simulink model "snap2_f_200msps_64i_4096c"  (R2019a)
settings: Solver=VariableStepDiscrete  StartTime=0.0  StopTime=10.0  RelTol=1e-3
undefined symbols (not defined in the file or in its folder): datetime, posixtime
libraries: xbsIndex_r4 x21354, casper_library_misc x297, casper_library_delays x19, xps_library x14, casper_library_sources x4
(part 28 of 217)

== system snap2_f_200msps_64i_4096c/input/rms ==
  note: two clocks after
      | adc_rms_rst goes high
      | the outputs are locked
  note: To provide a means for measuring the magnitude of the signals
      | coming in to each ADC channel, we have a "calc_adc_sum_sq"
      | block which uses a single multiplier, two accumulators, and two
      | regsiters to calculate the sum of 64K ADC samples and the sum
      | of squares of 64K ADC samples.  These can be used to calculate
      | the mean (aka DC offset) and standard deviation (aka RMS) of
      | the ADC inputs.
  note: The sum_sumsq values are Fix_64_0.
      | The upper 29 bits are Fix_29_0 sum of samples.
      | The lower 35 bits are UFix_35_0 sum of squares.
  note: sum,sq,sum,sq,...
  in : Inport
  Constant : Constant  Value=0
  Counter : xbsIndex_r4/Counter  cnt_type=Free Running  cnt_to=Inf  operation=Up  start_count=0  cnt_by_val=1  arith_type=Unsigned  n_bits=16  bin_pt=0  load_pin=off  rst=off  en=off  explicit_period=off  period=1  use_behavioral_HDL=off  implementation=Fabric  use_rpm=on  dbl_ovrd=off  block_type=counter
      settings: xl_area=[0, 0, 0, 0, 0, 0, 0]
  Slice16 : xbsIndex_r4/Slice  nbits=1  boolean_output=on  mode=Upper Bit Location + Width  bit1=0  base1=MSB of Input  bit0=19  base0=LSB of Input  dbl_ovrd=off  block_type=slice
      settings: infoedit="Extracts a given range of bits from each input sample and presents it at the output.  The output type is ordinarily unsigned with binary point at zero, but can be Boolean when the slice is one bit wide.<P><P>Hardware notes: In hardware this block costs nothing."  block_version=10.1.3
  Terminator : Terminator
  bram_ctrl : Subsystem
  bus_expand : Subsystem  AncestorBlock=casper_library_flow_control/bus_expand  mask(bus_expand){mode=divisions of equal size, outputNum=64, outputWidth=10, outputBinaryPt=0, outputArithmeticType=1, show_format=off, outputToWorkspace=off, variablePrefix=out, outputToModelAsWell=on}
      mask prompts: outputNum "Number of outputs:"; outputWidth "Output width:"; outputBinaryPt "Output binary point position:"; outputArithmeticType "Output arithmetic type (ufix=0, fix=1, bool=2):"; show_format "Print format string?"; outputToWorkspace "Output to workspace?"; variablePrefix "Variable name prefix:"; outputToModelAsWell "Output to model as well?"
      mask help:
      | Expands a 'bus' made using a bus_create or Xilinx
      | concat block.
      | The input will be divided into the specified number
      | of outputs with the specified arithmetic types.
      | Divisions are made from most significant bit.
      mask init: same as snap2_f_200msps_64i_4096c/autocorr/bus_expand
      settings: AttributesFormatString=64 outputs
      mask TypeOptions mode: divisions of equal size | divisions of arbitrary size
      mask Callback mode: bus_expand_callback();
      mask Callback outputWidth: bus_expand_callback();
      mask Callback outputToWorkspace: bus_expand_callback();
  calc_adc_sum_sq0 : Subsystem
  calc_adc_sum_sq1 : Subsystem
  calc_adc_sum_sq10 : Subsystem
  calc_adc_sum_sq11 : Subsystem
  calc_adc_sum_sq12 : Subsystem
  calc_adc_sum_sq13 : Subsystem
  calc_adc_sum_sq14 : Subsystem
  calc_adc_sum_sq15 : Subsystem
  calc_adc_sum_sq16 : Subsystem
  calc_adc_sum_sq17 : Subsystem
  calc_adc_sum_sq18 : Subsystem
  calc_adc_sum_sq19 : Subsystem
  calc_adc_sum_sq2 : Subsystem
  calc_adc_sum_sq20 : Subsystem
  calc_adc_sum_sq21 : Subsystem
  calc_adc_sum_sq22 : Subsystem
  calc_adc_sum_sq23 : Subsystem
  calc_adc_sum_sq24 : Subsystem
  calc_adc_sum_sq25 : Subsystem
  calc_adc_sum_sq26 : Subsystem
  calc_adc_sum_sq27 : Subsystem
  calc_adc_sum_sq28 : Subsystem
  calc_adc_sum_sq29 : Subsystem
  calc_adc_sum_sq3 : Subsystem
  calc_adc_sum_sq30 : Subsystem
  calc_adc_sum_sq31 : Subsystem
  calc_adc_sum_sq32 : Subsystem
  calc_adc_sum_sq33 : Subsystem
  calc_adc_sum_sq34 : Subsystem
  calc_adc_sum_sq35 : Subsystem
  calc_adc_sum_sq36 : Subsystem
  calc_adc_sum_sq37 : Subsystem
  calc_adc_sum_sq38 : Subsystem
  calc_adc_sum_sq39 : Subsystem
  calc_adc_sum_sq4 : Subsystem
  calc_adc_sum_sq40 : Subsystem
  calc_adc_sum_sq41 : Subsystem
  calc_adc_sum_sq42 : Subsystem
  calc_adc_sum_sq43 : Subsystem
  calc_adc_sum_sq44 : Subsystem
  calc_adc_sum_sq45 : Subsystem
  calc_adc_sum_sq46 : Subsystem
  calc_adc_sum_sq47 : Subsystem
  calc_adc_sum_sq48 : Subsystem
  calc_adc_sum_sq49 : Subsystem
  calc_adc_sum_sq5 : Subsystem
  calc_adc_sum_sq50 : Subsystem
  calc_adc_sum_sq51 : Subsystem
  calc_adc_sum_sq52 : Subsystem
  calc_adc_sum_sq53 : Subsystem
  calc_adc_sum_sq54 : Subsystem
  calc_adc_sum_sq55 : Subsystem
  calc_adc_sum_sq56 : Subsystem
  calc_adc_sum_sq57 : Subsystem
  calc_adc_sum_sq58 : Subsystem
  calc_adc_sum_sq59 : Subsystem
  calc_adc_sum_sq6 : Subsystem
  calc_adc_sum_sq60 : Subsystem
  calc_adc_sum_sq61 : Subsystem
  calc_adc_sum_sq62 : Subsystem
  calc_adc_sum_sq63 : Subsystem
  calc_adc_sum_sq7 : Subsystem
  calc_adc_sum_sq8 : Subsystem
  calc_adc_sum_sq9 : Subsystem
  edge_detect : Subsystem  AncestorBlock=casper_library_misc/edge_detect  mask(edge_detect){edge=Rising, polarity=Active High, x_in=[0 0.08 0.08 0.16 0.16 0.24 0.24 0.32 0.32 0.4], y_in=[-1 -1  1  1  1  1  1  1  1  1], x_out=[0.6 0.68 0.68 0.76 0.76 0.84 0.84 0.92 0.92 1], y_out=[-1 -1  1  1 -1 -1 -1 -1 -1 -1]}
      mask prompts: edge "Edge Type"; polarity "Output Polarity"; x_in "Input X Positions"; y_in "Input Y Positions"; x_out "Output X Positions"; y_out "Output Y Positions"
      mask help: Output is active for one-cycle after each edge of the specified type (i.e. rising, falling or both).
      mask init: same as snap2_f_200msps_64i_4096c/cosmic_ray/edge_detect
      settings: AttributesFormatString=|
      | rising edges
      | active high
      mask Help: Output is active for one-cycle after each edge of the specified type (i.e. rising, falling, or both).  Latency is zero.
      mask TypeOptions edge: Rising | Falling | Both
      mask TypeOptions polarity: Active High | Active Low
      mask Display:
      | plot(x_in_num,0.5+y_in_num*0.2);
      | plot(x_out_num,0.5+y_out_num*0.2);
  enable : Subsystem  Tag=xps:sw_reg  AncestorBlock=xps_library/Memory/software_register  mask(swreg){io_dir=From Processor, io_delay=0, init_val=0, sample_period=1, names=reg, bitwidths=32, bin_pts=0, arith_types=0, sim_port=on, show_format=off, desc_str=|}
      mask desc_str=|
      | Enable statistics recording. If the least-significant bit
      | is ``1``, statistics will be recorded to RAM.
      mask prompts: io_dir "I/O direction"; io_delay "I/O delay"; init_val "Initial Value"; sample_period "Sample period"; names "Bitfield names [msb...lsb]"; bitwidths "Bitfield widths"; bin_pts "Bitfield binary pts"; arith_types "Bitfield types, ufix=0, fix=1, bool=2"; sim_port "Provide sim input/output?"; show_format "Print format string?"; desc_str "Description"
      mask help: A 32-bit software-accessible register. Can be divided into bitfields of varying widths and types using the fields in the block mask.
      mask init:
      | swreg_init(gcb)
      settings: AttributesFormatString=1input
      mask TypeOptions io_dir: To Processor | From Processor
      mask Callback io_dir:
      | mask_enables = get_param(gcb, 'MaskEnables');
      | mask_names = get_param(gcb, 'MaskNames');
      | if strcmp(get_param(gcb, 'io_dir'), 'To Processor'),
      |     mask_enables{ismember(mask_names, 'sample_period')} = 'off';
      | else
      |     mask_enables{ismember(mask_names, 'sample_period')} = 'on';
      | end
      | set_param(gcb, 'MaskEnables', mask_enables);
      mask DialogControl ParameterTabVar0 Prompt: Setup
  levels : Subsystem  Tag=xps:bram  AncestorBlock=xps_library/Memory/shared_bram  mask{sample_rate=1, init_vals=[0:2^10-1], data_bin_pt=0, optimization=Minimum_Area, reg_core_output=on, reg_prim_output=on, data_width=64, addr_width=9, arith_type=Unsigned, desc_str=|, type_desc=uint64}
      mask desc_str=|
      | Multi-channel statistics. For the ``n`` th 64-bit word, the
      | least signficant 32 bits represent the accumulated
      | ADC power, accumulated over 65536 samples and
      | stored as an unsigned 32-bit integer.
      | The most significant 32 bits represent the sum of
      | 65536 ADC samples stored as a signed 32-bit integer.
      mask prompts: sample_rate "Sample rate"; init_vals "Initial values (simulation only)"; data_bin_pt "Data Binary Point"; reg_core_output "Register Core Output"; reg_prim_output "Register Primitive Output"; data_width "Data Width"; addr_width "Address width"; arith_type "Output Data Type"; desc_str "Description"; type_desc "Word Type Description"
      mask init:
      | shared_bram_mask;
      mask TypeOptions optimization: Minimum_Area | Low_Power
      mask TypeOptions data_width: 8 | 16 | 32 | 64 | 128
      mask TypeOptions arith_type: Unsigned | Signed  (2's comp)
      mask DialogControl Container4 Prompt: Configuration
      mask DialogControl Container10 Prompt: Documentation
  lsb : xbsIndex_r4/Slice  nbits=0  boolean_output=on  mode=Lower Bit Location + Width  bit1=0  base1=MSB of Input  bit0=0  base0=LSB of Input  dbl_ovrd=off  block_type=slice
      settings: block_version=10.1.3
  tag scope: adc_rms_rst=global
  wires:
  Counter/1 -> Slice16/1
  Slice16/1 -> edge_detect/1(in)
  edge_detect/1(out) -> [adc_rms_rst]
  enable/1(in_reg) -> lsb/1
  bram_ctrl/1(addr) -> levels/1(addr)
  bram_ctrl/2(data) -> levels/2(data_in)
  bram_ctrl/3(we) -> levels/3(we)
  Constant/1 -> enable/1(sim_1)
  levels/1(data_out) -> Terminator/1
  in/1 -> bus_expand/1(bus_in)
  lsb/1 -> bram_ctrl/1(en)
  calc_adc_sum_sq36/1(sum_sumsq) -> bram_ctrl/46(adc44)
  calc_adc_sum_sq12/1(sum_sumsq) -> bram_ctrl/14(adc12)
  calc_adc_sum_sq30/1(sum_sumsq) -> bram_ctrl/26(adc24)
  calc_adc_sum_sq28/1(sum_sumsq) -> bram_ctrl/24(adc22)
  calc_adc_sum_sq58/1(sum_sumsq) -> bram_ctrl/38(adc36)
  calc_adc_sum_sq55/1(sum_sumsq) -> bram_ctrl/37(adc35)
  calc_adc_sum_sq18/1(sum_sumsq) -> bram_ctrl/28(adc26)
  calc_adc_sum_sq24/1(sum_sumsq) -> bram_ctrl/20(adc18)
  calc_adc_sum_sq22/1(sum_sumsq) -> bram_ctrl/32(adc30)
  calc_adc_sum_sq32/1(sum_sumsq) -> bram_ctrl/34(adc32)
  calc_adc_sum_sq25/1(sum_sumsq) -> bram_ctrl/21(adc19)
  calc_adc_sum_sq23/1(sum_sumsq) -> bram_ctrl/33(adc31)
  calc_adc_sum_sq31/1(sum_sumsq) -> bram_ctrl/27(adc25)
  calc_adc_sum_sq19/1(sum_sumsq) -> bram_ctrl/29(adc27)
  calc_adc_sum_sq13/1(sum_sumsq) -> bram_ctrl/15(adc13)
  calc_adc_sum_sq35/1(sum_sumsq) -> bram_ctrl/45(adc43)
  calc_adc_sum_sq39/1(sum_sumsq) -> bram_ctrl/49(adc47)
  calc_adc_sum_sq38/1(sum_sumsq) -> bram_ctrl/48(adc46)
  calc_adc_sum_sq57/1(sum_sumsq) -> bram_ctrl/59(adc57)
  calc_adc_sum_sq48/1(sum_sumsq) -> bram_ctrl/65(adc63)
  calc_adc_sum_sq16/1(sum_sumsq) -> bram_ctrl/18(adc16)
  calc_adc_sum_sq27/1(sum_sumsq) -> bram_ctrl/23(adc21)
  calc_adc_sum_sq50/1(sum_sumsq) -> bram_ctrl/53(adc51)
  calc_adc_sum_sq42/1(sum_sumsq) -> bram_ctrl/60(adc58)
  calc_adc_sum_sq15/1(sum_sumsq) -> bram_ctrl/17(adc15)
  calc_adc_sum_sq26/1(sum_sumsq) -> bram_ctrl/22(adc20)
  calc_adc_sum_sq49/1(sum_sumsq) -> bram_ctrl/52(adc50)
  calc_adc_sum_sq54/1(sum_sumsq) -> bram_ctrl/57(adc55)
  calc_adc_sum_sq51/1(sum_sumsq) -> bram_ctrl/54(adc52)
  calc_adc_sum_sq14/1(sum_sumsq) -> bram_ctrl/16(adc14)
  calc_adc_sum_sq20/1(sum_sumsq) -> bram_ctrl/30(adc28)
  calc_adc_sum_sq17/1(sum_sumsq) -> bram_ctrl/19(adc17)
  calc_adc_sum_sq33/1(sum_sumsq) -> bram_ctrl/35(adc33)
  calc_adc_sum_sq53/1(sum_sumsq) -> bram_ctrl/56(adc54)
  calc_adc_sum_sq21/1(sum_sumsq) -> bram_ctrl/31(adc29)
  calc_adc_sum_sq59/1(sum_sumsq) -> bram_ctrl/39(adc37)
  calc_adc_sum_sq47/1(sum_sumsq) -> bram_ctrl/64(adc62)
  calc_adc_sum_sq52/1(sum_sumsq) -> bram_ctrl/55(adc53)
  calc_adc_sum_sq61/1(sum_sumsq) -> bram_ctrl/41(adc39)
  calc_adc_sum_sq46/1(sum_sumsq) -> bram_ctrl/63(adc61)
  calc_adc_sum_sq34/1(sum_sumsq) -> bram_ctrl/44(adc42)
  calc_adc_sum_sq56/1(sum_sumsq) -> bram_ctrl/58(adc56)
  calc_adc_sum_sq60/1(sum_sumsq) -> bram_ctrl/40(adc38)
  calc_adc_sum_sq62/1(sum_sumsq) -> bram_ctrl/42(adc40)
  calc_adc_sum_sq29/1(sum_sumsq) -> bram_ctrl/25(adc23)
  calc_adc_sum_sq44/1(sum_sumsq) -> bram_ctrl/36(adc34)
  calc_adc_sum_sq41/1(sum_sumsq) -> bram_ctrl/51(adc49)
  calc_adc_sum_sq37/1(sum_sumsq) -> bram_ctrl/47(adc45)
  calc_adc_sum_sq43/1(sum_sumsq) -> bram_ctrl/61(adc59)
  calc_adc_sum_sq63/1(sum_sumsq) -> bram_ctrl/43(adc41)
  calc_adc_sum_sq40/1(sum_sumsq) -> bram_ctrl/50(adc48)
  calc_adc_sum_sq0/1(sum_sumsq) -> bram_ctrl/2(adc0)
  calc_adc_sum_sq1/1(sum_sumsq) -> bram_ctrl/3(adc1)
  calc_adc_sum_sq10/1(sum_sumsq) -> bram_ctrl/12(adc10)
  calc_adc_sum_sq11/1(sum_sumsq) -> bram_ctrl/13(adc11)
  calc_adc_sum_sq2/1(sum_sumsq) -> bram_ctrl/4(adc2)
  calc_adc_sum_sq3/1(sum_sumsq) -> bram_ctrl/5(adc3)
  calc_adc_sum_sq4/1(sum_sumsq) -> bram_ctrl/6(adc4)
  calc_adc_sum_sq5/1(sum_sumsq) -> bram_ctrl/7(adc5)
  calc_adc_sum_sq6/1(sum_sumsq) -> bram_ctrl/8(adc6)
  calc_adc_sum_sq7/1(sum_sumsq) -> bram_ctrl/9(adc7)
  calc_adc_sum_sq8/1(sum_sumsq) -> bram_ctrl/10(adc8)
  calc_adc_sum_sq9/1(sum_sumsq) -> bram_ctrl/11(adc9)
  calc_adc_sum_sq45/1(sum_sumsq) -> bram_ctrl/62(adc60)
  bus_expand/41(out24) -> calc_adc_sum_sq62/1(in)
  bus_expand/40(out25) -> calc_adc_sum_sq61/1(in)
  bus_expand/39(out26) -> calc_adc_sum_sq60/1(in)
  bus_expand/1(msb_out64) -> calc_adc_sum_sq0/1(in)
  bus_expand/2(out63) -> calc_adc_sum_sq1/1(in)
  bus_expand/45(out20) -> calc_adc_sum_sq36/1(in)
  bus_expand/30(out35) -> calc_adc_sum_sq21/1(in)
  bus_expand/33(out32) -> calc_adc_sum_sq32/1(in)
  bus_expand/52(out13) -> calc_adc_sum_sq50/1(in)
  bus_expand/35(out30) -> calc_adc_sum_sq44/1(in)
  bus_expand/51(out14) -> calc_adc_sum_sq49/1(in)
  bus_expand/49(out16) -> calc_adc_sum_sq40/1(in)
  bus_expand/44(out21) -> calc_adc_sum_sq35/1(in)
  bus_expand/53(out12) -> calc_adc_sum_sq51/1(in)
  bus_expand/5(out60) -> calc_adc_sum_sq4/1(in)
  bus_expand/7(out58) -> calc_adc_sum_sq6/1(in)
  bus_expand/4(out61) -> calc_adc_sum_sq3/1(in)
  bus_expand/37(out28) -> calc_adc_sum_sq58/1(in)
  bus_expand/9(out56) -> calc_adc_sum_sq8/1(in)
  bus_expand/10(out55) -> calc_adc_sum_sq9/1(in)
  bus_expand/11(out54) -> calc_adc_sum_sq10/1(in)
  bus_expand/34(out31) -> calc_adc_sum_sq33/1(in)
  bus_expand/36(out29) -> calc_adc_sum_sq55/1(in)
  bus_expand/48(out17) -> calc_adc_sum_sq39/1(in)
  bus_expand/29(out36) -> calc_adc_sum_sq20/1(in)
  bus_expand/47(out18) -> calc_adc_sum_sq38/1(in)
  bus_expand/31(out34) -> calc_adc_sum_sq22/1(in)
  bus_expand/43(out22) -> calc_adc_sum_sq34/1(in)
  bus_expand/50(out15) -> calc_adc_sum_sq41/1(in)
  bus_expand/46(out19) -> calc_adc_sum_sq37/1(in)
  bus_expand/38(out27) -> calc_adc_sum_sq59/1(in)
  bus_expand/17(out48) -> calc_adc_sum_sq16/1(in)
  bus_expand/13(out52) -> calc_adc_sum_sq12/1(in)
  bus_expand/14(out51) -> calc_adc_sum_sq13/1(in)
  bus_expand/15(out50) -> calc_adc_sum_sq14/1(in)
  bus_expand/16(out49) -> calc_adc_sum_sq15/1(in)
  bus_expand/18(out47) -> calc_adc_sum_sq17/1(in)
  bus_expand/19(out46) -> calc_adc_sum_sq24/1(in)
  bus_expand/20(out45) -> calc_adc_sum_sq25/1(in)
  bus_expand/21(out44) -> calc_adc_sum_sq26/1(in)
  bus_expand/22(out43) -> calc_adc_sum_sq27/1(in)
  bus_expand/23(out42) -> calc_adc_sum_sq28/1(in)
  bus_expand/24(out41) -> calc_adc_sum_sq29/1(in)
  bus_expand/25(out40) -> calc_adc_sum_sq30/1(in)
  bus_expand/26(out39) -> calc_adc_sum_sq31/1(in)
  bus_expand/27(out38) -> calc_adc_sum_sq18/1(in)
  bus_expand/28(out37) -> calc_adc_sum_sq19/1(in)
  bus_expand/3(out62) -> calc_adc_sum_sq2/1(in)
  bus_expand/8(out57) -> calc_adc_sum_sq7/1(in)
  bus_expand/12(out53) -> calc_adc_sum_sq11/1(in)
  bus_expand/6(out59) -> calc_adc_sum_sq5/1(in)
  bus_expand/42(out23) -> calc_adc_sum_sq63/1(in)
  bus_expand/32(out33) -> calc_adc_sum_sq23/1(in)
  bus_expand/54(out11) -> calc_adc_sum_sq52/1(in)
  bus_expand/55(out10) -> calc_adc_sum_sq53/1(in)
  bus_expand/56(out9) -> calc_adc_sum_sq54/1(in)
  bus_expand/57(out8) -> calc_adc_sum_sq56/1(in)
  bus_expand/58(out7) -> calc_adc_sum_sq57/1(in)
  bus_expand/59(out6) -> calc_adc_sum_sq42/1(in)
  bus_expand/60(out5) -> calc_adc_sum_sq43/1(in)
  bus_expand/61(out4) -> calc_adc_sum_sq45/1(in)
  bus_expand/62(out3) -> calc_adc_sum_sq46/1(in)
  bus_expand/63(out2) -> calc_adc_sum_sq47/1(in)
  bus_expand/64(lsb_out1) -> calc_adc_sum_sq48/1(in)

== system snap2_f_200msps_64i_4096c/input/source_sel0 ==
  sim_1 : Inport
  convert1_1 : DataTypeConversion  OutDataTypeStr=fixdt('ufix32_En0')  LockScale=on
  convert2_1 : DataTypeConversion  OutDataTypeStr=fixdt('ufix32_En0')  ConvertRealWorld=Stored Integer (SI)  LockScale=on
  gain_1 : Gain
  io_delay : xbsIndex_r4/Delay  rst=off  infoeditControl=Selection of Reset will increase slice count due to use of real FFs and instead of SRLs  en=off  latency=0  reg_retiming=on  dbl_ovrd=off  block_type=delay
  reint1 : xbsIndex_r4/Reinterpret  force_arith_type=on  arith_type=Unsigned  force_bin_pt=on  bin_pt=0  block_type=reinterpret
  slice_reg : xbsIndex_r4/Slice  nbits=32  boolean_output=off  mode=Lower Bit Location + Width  bit1=0  base1=MSB of Input  bit0=0  base0=LSB of Input  dbl_ovrd=off  block_type=slice
  snap2_f_200msps_64i_4096c_input_source_sel0_user_data_out : xbsIndex_r4/Gateway In  gui_display_data_type=Fixed-point  arith_type=Unsigned  n_bits=32  bin_pt=0  preci_type=Single  exp_width=8  frac_width=24  rows=1  columns=1  quantization="Round  (unbiased: +/- Inf)"  overflow=Saturate  period=1  UseAsADC=off  ADCChannel='1'  interface=None  automatic_assignment=on  address_offset=hex2dec('00')  intf_name=''  intf_description=''  default_value=0  timing_constraint=None  locs_specified=off  LOCs={}  io_standard={}  inherit_from_input=off  hdl_port=on  dbl_ovrd=off  block_type=gatewayin
  in_reg : Outport
  wires:
  snap2_f_200msps_64i_4096c_input_source_sel0_user_data_out/1 -> io_delay/1
  sim_1/1 -> convert1_1/1
  convert1_1/1 -> convert2_1/1
  convert2_1/1 -> gain_1/1
  gain_1/1 -> snap2_f_200msps_64i_4096c_input_source_sel0_user_data_out/1
  io_delay/1 -> slice_reg/1
  slice_reg/1 -> reint1/1
  reint1/1 -> in_reg/1

== system snap2_f_200msps_64i_4096c/input/source_sel1 ==
  sim_1 : Inport
  convert1_1 : DataTypeConversion  OutDataTypeStr=fixdt('ufix32_En0')  LockScale=on
  convert2_1 : DataTypeConversion  OutDataTypeStr=fixdt('ufix32_En0')  ConvertRealWorld=Stored Integer (SI)  LockScale=on
  gain_1 : Gain
  io_delay : xbsIndex_r4/Delay  rst=off  infoeditControl=Selection of Reset will increase slice count due to use of real FFs and instead of SRLs  en=off  latency=0  reg_retiming=on  dbl_ovrd=off  block_type=delay
  reint1 : xbsIndex_r4/Reinterpret  force_arith_type=on  arith_type=Unsigned  force_bin_pt=on  bin_pt=0  block_type=reinterpret
  slice_reg : xbsIndex_r4/Slice  nbits=32  boolean_output=off  mode=Lower Bit Location + Width  bit1=0  base1=MSB of Input  bit0=0  base0=LSB of Input  dbl_ovrd=off  block_type=slice
  snap2_f_200msps_64i_4096c_input_source_sel1_user_data_out : xbsIndex_r4/Gateway In  gui_display_data_type=Fixed-point  arith_type=Unsigned  n_bits=32  bin_pt=0  preci_type=Single  exp_width=8  frac_width=24  rows=1  columns=1  quantization="Round  (unbiased: +/- Inf)"  overflow=Saturate  period=1  UseAsADC=off  ADCChannel='1'  interface=None  automatic_assignment=on  address_offset=hex2dec('00')  intf_name=''  intf_description=''  default_value=0  timing_constraint=None  locs_specified=off  LOCs={}  io_standard={}  inherit_from_input=off  hdl_port=on  dbl_ovrd=off  block_type=gatewayin
  in_reg : Outport
  wires:
  snap2_f_200msps_64i_4096c_input_source_sel1_user_data_out/1 -> io_delay/1
  sim_1/1 -> convert1_1/1
  convert1_1/1 -> convert2_1/1
  convert2_1/1 -> gain_1/1
  gain_1/1 -> snap2_f_200msps_64i_4096c_input_source_sel1_user_data_out/1
  io_delay/1 -> slice_reg/1
  slice_reg/1 -> reint1/1
  reint1/1 -> in_reg/1

== system snap2_f_200msps_64i_4096c/input/source_sel2 ==
  sim_1 : Inport
  convert1_1 : DataTypeConversion  OutDataTypeStr=fixdt('ufix32_En0')  LockScale=on
  convert2_1 : DataTypeConversion  OutDataTypeStr=fixdt('ufix32_En0')  ConvertRealWorld=Stored Integer (SI)  LockScale=on
  gain_1 : Gain
  io_delay : xbsIndex_r4/Delay  rst=off  infoeditControl=Selection of Reset will increase slice count due to use of real FFs and instead of SRLs  en=off  latency=0  reg_retiming=on  dbl_ovrd=off  block_type=delay
  reint1 : xbsIndex_r4/Reinterpret  force_arith_type=on  arith_type=Unsigned  force_bin_pt=on  bin_pt=0  block_type=reinterpret
  slice_reg : xbsIndex_r4/Slice  nbits=32  boolean_output=off  mode=Lower Bit Location + Width  bit1=0  base1=MSB of Input  bit0=0  base0=LSB of Input  dbl_ovrd=off  block_type=slice
  snap2_f_200msps_64i_4096c_input_source_sel2_user_data_out : xbsIndex_r4/Gateway In  gui_display_data_type=Fixed-point  arith_type=Unsigned  n_bits=32  bin_pt=0  preci_type=Single  exp_width=8  frac_width=24  rows=1  columns=1  quantization="Round  (unbiased: +/- Inf)"  overflow=Saturate  period=1  UseAsADC=off  ADCChannel='1'  interface=None  automatic_assignment=on  address_offset=hex2dec('00')  intf_name=''  intf_description=''  default_value=0  timing_constraint=None  locs_specified=off  LOCs={}  io_standard={}  inherit_from_input=off  hdl_port=on  dbl_ovrd=off  block_type=gatewayin
  in_reg : Outport
  wires:
  snap2_f_200msps_64i_4096c_input_source_sel2_user_data_out/1 -> io_delay/1
  sim_1/1 -> convert1_1/1
  convert1_1/1 -> convert2_1/1
  convert2_1/1 -> gain_1/1
  gain_1/1 -> snap2_f_200msps_64i_4096c_input_source_sel2_user_data_out/1
  io_delay/1 -> slice_reg/1
  slice_reg/1 -> reint1/1
  reint1/1 -> in_reg/1

== system snap2_f_200msps_64i_4096c/input/source_sel3 ==
  sim_1 : Inport
  convert1_1 : DataTypeConversion  OutDataTypeStr=fixdt('ufix32_En0')  LockScale=on
  convert2_1 : DataTypeConversion  OutDataTypeStr=fixdt('ufix32_En0')  ConvertRealWorld=Stored Integer (SI)  LockScale=on
  gain_1 : Gain
  io_delay : xbsIndex_r4/Delay  rst=off  infoeditControl=Selection of Reset will increase slice count due to use of real FFs and instead of SRLs  en=off  latency=0  reg_retiming=on  dbl_ovrd=off  block_type=delay
  reint1 : xbsIndex_r4/Reinterpret  force_arith_type=on  arith_type=Unsigned  force_bin_pt=on  bin_pt=0  block_type=reinterpret
  slice_reg : xbsIndex_r4/Slice  nbits=32  boolean_output=off  mode=Lower Bit Location + Width  bit1=0  base1=MSB of Input  bit0=0  base0=LSB of Input  dbl_ovrd=off  block_type=slice
  snap2_f_200msps_64i_4096c_input_source_sel3_user_data_out : xbsIndex_r4/Gateway In  gui_display_data_type=Fixed-point  arith_type=Unsigned  n_bits=32  bin_pt=0  preci_type=Single  exp_width=8  frac_width=24  rows=1  columns=1  quantization="Round  (unbiased: +/- Inf)"  overflow=Saturate  period=1  UseAsADC=off  ADCChannel='1'  interface=None  automatic_assignment=on  address_offset=hex2dec('00')  intf_name=''  intf_description=''  default_value=0  timing_constraint=None  locs_specified=off  LOCs={}  io_standard={}  inherit_from_input=off  hdl_port=on  dbl_ovrd=off  block_type=gatewayin
  in_reg : Outport
  wires:
  snap2_f_200msps_64i_4096c_input_source_sel3_user_data_out/1 -> io_delay/1
  sim_1/1 -> convert1_1/1
  convert1_1/1 -> convert2_1/1
  convert2_1/1 -> gain_1/1
  gain_1/1 -> snap2_f_200msps_64i_4096c_input_source_sel3_user_data_out/1
  io_delay/1 -> slice_reg/1
  slice_reg/1 -> reint1/1
  reint1/1 -> in_reg/1

== system snap2_f_200msps_64i_4096c/mask/acc_cnt ==
  out_reg : Inport
  assert_reg : xbsIndex_r4/Assert  assert_type=on  type_source=Explicitly  gui_display_data_type=Fixed-point  arith_type=Unsigned  n_bits=32  bin_pt=0  preci_type=Single  exp_width=8  frac_width=24  assert_rate=off  rate_source=Explicitly  period=1  output_port=on  block_type=assert
  cast_gw : xbsIndex_r4/Convert  gui_display_data_type=Fixed-point  arith_type=Unsigned  n_bits=32  bin_pt=0  float_type=Single  exp_bits=8  fraction_bits=24  quantization=Truncate  overflow=Wrap  en=off  latency=1  pipeline=off  dbl_ovrd=off  block_type=convert
  io_delay : xbsIndex_r4/Delay  rst=off  infoeditControl=Selection of Reset will increase slice count due to use of real FFs and instead of SRLs  en=off  latency=0  reg_retiming=on  dbl_ovrd=off  block_type=delay
  reint1 : xbsIndex_r4/Reinterpret  force_arith_type=on  arith_type=Unsigned  force_bin_pt=on  bin_pt=0  block_type=reinterpret
  sim_out : Terminator
  sim_out_reg_gw : xbsIndex_r4/Gateway Out  inherit_from_input=off  hdl_port=off  rows=1  columns=1  UseAsDAC=off  DACChannel='1'  interface=None  automatic_assignment=on  address_offset=hex2dec('00')  intf_name=''  intf_description=''  timing_constraint=None  locs_specified=off  LOCs={}  io_standard={}  block_type=gatewayout
  sim_out_reg_sim_delay : xbsIndex_r4/Delay  rst=off  infoeditControl=Selection of Reset will increase slice count due to use of real FFs and instead of SRLs  en=off  latency=1  reg_retiming=on  dbl_ovrd=off  block_type=delay
  snap2_f_200msps_64i_4096c_mask_acc_cnt_user_data_in : xbsIndex_r4/Gateway Out  inherit_from_input=off  hdl_port=on  rows=1  columns=1  UseAsDAC=off  DACChannel='1'  interface=None  automatic_assignment=on  address_offset=hex2dec('00')  intf_name=''  intf_description=''  timing_constraint=None  locs_specified=off  LOCs={}  io_standard={}  block_type=gatewayout
  sim_out_reg : Outport
  wires:
  sim_out_reg_sim_delay/1 -> sim_out_reg_gw/1
  sim_out_reg_gw/1 -> sim_out_reg/1
  io_delay/1 -> cast_gw/1
  cast_gw/1 -> snap2_f_200msps_64i_4096c_mask_acc_cnt_user_data_in/1
  snap2_f_200msps_64i_4096c_mask_acc_cnt_user_data_in/1 -> sim_out/1
  out_reg/1 -> sim_out_reg_sim_delay/1, assert_reg/1
  assert_reg/1 -> reint1/1
  reint1/1 -> io_delay/1

== system snap2_f_200msps_64i_4096c/mask/acc_len ==
  sim_1 : Inport
  convert1_1 : DataTypeConversion  OutDataTypeStr=fixdt('ufix32_En0')  LockScale=on
  convert2_1 : DataTypeConversion  OutDataTypeStr=fixdt('ufix32_En0')  ConvertRealWorld=Stored Integer (SI)  LockScale=on
  gain_1 : Gain
  io_delay : xbsIndex_r4/Delay  rst=off  infoeditControl=Selection of Reset will increase slice count due to use of real FFs and instead of SRLs  en=off  latency=0  reg_retiming=on  dbl_ovrd=off  block_type=delay
  reint1 : xbsIndex_r4/Reinterpret  force_arith_type=on  arith_type=Unsigned  force_bin_pt=on  bin_pt=0  block_type=reinterpret
  slice_reg : xbsIndex_r4/Slice  nbits=32  boolean_output=off  mode=Lower Bit Location + Width  bit1=0  base1=MSB of Input  bit0=0  base0=LSB of Input  dbl_ovrd=off  block_type=slice
  snap2_f_200msps_64i_4096c_mask_acc_len_user_data_out : xbsIndex_r4/Gateway In  gui_display_data_type=Fixed-point  arith_type=Unsigned  n_bits=32  bin_pt=0  preci_type=Single  exp_width=8  frac_width=24  rows=1  columns=1  quantization="Round  (unbiased: +/- Inf)"  overflow=Saturate  period=1  UseAsADC=off  ADCChannel='1'  interface=None  automatic_assignment=on  address_offset=hex2dec('00')  intf_name=''  intf_description=''  default_value=0  timing_constraint=None  locs_specified=off  LOCs={}  io_standard={}  inherit_from_input=off  hdl_port=on  dbl_ovrd=off  block_type=gatewayin
  in_reg : Outport
  wires:
  snap2_f_200msps_64i_4096c_mask_acc_len_user_data_out/1 -> io_delay/1
  sim_1/1 -> convert1_1/1
  convert1_1/1 -> convert2_1/1
  convert2_1/1 -> gain_1/1
  gain_1/1 -> snap2_f_200msps_64i_4096c_mask_acc_len_user_data_out/1
  io_delay/1 -> slice_reg/1
  slice_reg/1 -> reint1/1
  reint1/1 -> in_reg/1

== system snap2_f_200msps_64i_4096c/mask/acc_time_lsb ==
  out_reg : Inport
  assert_reg : xbsIndex_r4/Assert  assert_type=on  type_source=Explicitly  gui_display_data_type=Fixed-point  arith_type=Unsigned  n_bits=32  bin_pt=0  preci_type=Single  exp_width=8  frac_width=24  assert_rate=off  rate_source=Explicitly  period=1  output_port=on  block_type=assert
  cast_gw : xbsIndex_r4/Convert  gui_display_data_type=Fixed-point  arith_type=Unsigned  n_bits=32  bin_pt=0  float_type=Single  exp_bits=8  fraction_bits=24  quantization=Truncate  overflow=Wrap  en=off  latency=1  pipeline=off  dbl_ovrd=off  block_type=convert
  io_delay : xbsIndex_r4/Delay  rst=off  infoeditControl=Selection of Reset will increase slice count due to use of real FFs and instead of SRLs  en=off  latency=0  reg_retiming=on  dbl_ovrd=off  block_type=delay
  reint1 : xbsIndex_r4/Reinterpret  force_arith_type=on  arith_type=Unsigned  force_bin_pt=on  bin_pt=0  block_type=reinterpret
  sim_out : Terminator
  sim_out_reg_gw : xbsIndex_r4/Gateway Out  inherit_from_input=off  hdl_port=off  rows=1  columns=1  UseAsDAC=off  DACChannel='1'  interface=None  automatic_assignment=on  address_offset=hex2dec('00')  intf_name=''  intf_description=''  timing_constraint=None  locs_specified=off  LOCs={}  io_standard={}  block_type=gatewayout
  sim_out_reg_sim_delay : xbsIndex_r4/Delay  rst=off  infoeditControl=Selection of Reset will increase slice count due to use of real FFs and instead of SRLs  en=off  latency=1  reg_retiming=on  dbl_ovrd=off  block_type=delay
  snap2_f_200msps_64i_4096c_mask_acc_time_lsb_user_data_in : xbsIndex_r4/Gateway Out  inherit_from_input=off  hdl_port=on  rows=1  columns=1  UseAsDAC=off  DACChannel='1'  interface=None  automatic_assignment=on  address_offset=hex2dec('00')  intf_name=''  intf_description=''  timing_constraint=None  locs_specified=off  LOCs={}  io_standard={}  block_type=gatewayout
  sim_out_reg : Outport
  wires:
  sim_out_reg_sim_delay/1 -> sim_out_reg_gw/1
  sim_out_reg_gw/1 -> sim_out_reg/1
  io_delay/1 -> cast_gw/1
  cast_gw/1 -> snap2_f_200msps_64i_4096c_mask_acc_time_lsb_user_data_in/1
  snap2_f_200msps_64i_4096c_mask_acc_time_lsb_user_data_in/1 -> sim_out/1
  out_reg/1 -> sim_out_reg_sim_delay/1, assert_reg/1
  assert_reg/1 -> reint1/1
  reint1/1 -> io_delay/1

== system snap2_f_200msps_64i_4096c/mask/acc_time_msb ==
  out_reg : Inport
  assert_reg : xbsIndex_r4/Assert  assert_type=on  type_source=Explicitly  gui_display_data_type=Fixed-point  arith_type=Unsigned  n_bits=32  bin_pt=0  preci_type=Single  exp_width=8  frac_width=24  assert_rate=off  rate_source=Explicitly  period=1  output_port=on  block_type=assert
  cast_gw : xbsIndex_r4/Convert  gui_display_data_type=Fixed-point  arith_type=Unsigned  n_bits=32  bin_pt=0  float_type=Single  exp_bits=8  fraction_bits=24  quantization=Truncate  overflow=Wrap  en=off  latency=1  pipeline=off  dbl_ovrd=off  block_type=convert
  io_delay : xbsIndex_r4/Delay  rst=off  infoeditControl=Selection of Reset will increase slice count due to use of real FFs and instead of SRLs  en=off  latency=0  reg_retiming=on  dbl_ovrd=off  block_type=delay
  reint1 : xbsIndex_r4/Reinterpret  force_arith_type=on  arith_type=Unsigned  force_bin_pt=on  bin_pt=0  block_type=reinterpret
  sim_out : Terminator
  sim_out_reg_gw : xbsIndex_r4/Gateway Out  inherit_from_input=off  hdl_port=off  rows=1  columns=1  UseAsDAC=off  DACChannel='1'  interface=None  automatic_assignment=on  address_offset=hex2dec('00')  intf_name=''  intf_description=''  timing_constraint=None  locs_specified=off  LOCs={}  io_standard={}  block_type=gatewayout
  sim_out_reg_sim_delay : xbsIndex_r4/Delay  rst=off  infoeditControl=Selection of Reset will increase slice count due to use of real FFs and instead of SRLs  en=off  latency=1  reg_retiming=on  dbl_ovrd=off  block_type=delay
  snap2_f_200msps_64i_4096c_mask_acc_time_msb_user_data_in : xbsIndex_r4/Gateway Out  inherit_from_input=off  hdl_port=on  rows=1  columns=1  UseAsDAC=off  DACChannel='1'  interface=None  automatic_assignment=on  address_offset=hex2dec('00')  intf_name=''  intf_description=''  timing_constraint=None  locs_specified=off  LOCs={}  io_standard={}  block_type=gatewayout
  sim_out_reg : Outport
  wires:
  sim_out_reg_sim_delay/1 -> sim_out_reg_gw/1
  sim_out_reg_gw/1 -> sim_out_reg/1
  io_delay/1 -> cast_gw/1
  cast_gw/1 -> snap2_f_200msps_64i_4096c_mask_acc_time_msb_user_data_in/1
  snap2_f_200msps_64i_4096c_mask_acc_time_msb_user_data_in/1 -> sim_out/1
  out_reg/1 -> sim_out_reg_sim_delay/1, assert_reg/1
  assert_reg/1 -> reint1/1
  reint1/1 -> io_delay/1

== system snap2_f_200msps_64i_4096c/mask/bus_create2 ==
  in1 : Inport
  in2 : Inport  Port=2
  in3 : Inport  Port=3
  in4 : Inport  Port=4
  concatenate : xbsIndex_r4/Concat  num_inputs=4  dbl_ovrd=off  block_type=concat
  reinterpret{1..4} (4 alike) : xbsIndex_r4/Reinterpret  force_arith_type=on  arith_type=Unsigned  force_bin_pt=on  bin_pt=0  block_type=reinterpret
      reinterpret1 settings: infoedit="Changes signal type without altering the binary representation.   You can changed the signal between signed and unsigned, and relocate the binary point.<br><br>Hardware notes: In hardware this block costs nothing.<br><br>Example:  Suppose the input is 6 bits wide, signed, with 2 fractional bits, and the output is forced to unsigned with 0 fractional bits.  Then an input of -2.0 (1110.00 in binary 2's complement) becomes an output of 56 (111000 in binary)."
      reinterpret2 settings: infoedit="Changes signal type without altering the binary representation.   You can changed the signal between signed and unsigned, and relocate the binary point.<br><br>Hardware notes: In hardware this block costs nothing.<br><br>Example:  Suppose the input is 6 bits wide, signed, with 2 fractional bits, and the output is forced to unsigned with 0 fractional bits.  Then an input of -2.0 (1110.00 in binary 2's complement) becomes an output of 56 (111000 in binary)."
  bus_out : Outport
  wires:
  reinterpret4/1 -> concatenate/4
  in4/1 -> reinterpret4/1
  reinterpret3/1 -> concatenate/3
  in3/1 -> reinterpret3/1
  reinterpret2/1 -> concatenate/2
  in2/1 -> reinterpret2/1
  reinterpret1/1 -> concatenate/1
  in1/1 -> reinterpret1/1
  concatenate/1 -> bus_out/1

== system snap2_f_200msps_64i_4096c/mask/bus_expand ==
  bus_in : Inport
  reinterpret1 : xbsIndex_r4/Reinterpret  force_arith_type=on  arith_type=Unsigned  force_bin_pt=on  bin_pt=0  block_type=reinterpret
  reinterpret2 : xbsIndex_r4/Reinterpret  force_arith_type=on  arith_type=Unsigned  force_bin_pt=on  bin_pt=0  block_type=reinterpret
  slice1 : xbsIndex_r4/Slice  nbits=32  boolean_output=off  mode=Upper Bit Location + Width  bit1=-32  base1=MSB of Input  bit0=0  base0=LSB of Input  dbl_ovrd=off  block_type=slice
  slice2 : xbsIndex_r4/Slice  nbits=32  boolean_output=off  mode=Upper Bit Location + Width  bit1=0  base1=MSB of Input  bit0=0  base0=LSB of Input  dbl_ovrd=off  block_type=slice
  msb_out2 : Outport
  lsb_out1 : Outport  Port=2
  wires:
  bus_in/1 -> slice2/1, slice1/1
  slice2/1 -> reinterpret2/1
  reinterpret2/1 -> msb_out2/1
  slice1/1 -> reinterpret1/1
  reinterpret1/1 -> lsb_out1/1

== system snap2_f_200msps_64i_4096c/mask/bus_expand4 ==
  bus_in : Inport
  reinterpret{1..4} (4 alike) : xbsIndex_r4/Reinterpret  force_arith_type=on  arith_type=Unsigned  force_bin_pt=on  bin_pt=0  block_type=reinterpret
  slice1 : xbsIndex_r4/Slice  nbits=288  boolean_output=off  mode=Upper Bit Location + Width  bit1=-864  base1=MSB of Input  bit0=0  base0=LSB of Input  dbl_ovrd=off  block_type=slice
  slice2 : xbsIndex_r4/Slice  nbits=288  boolean_output=off  mode=Upper Bit Location + Width  bit1=-576  base1=MSB of Input  bit0=0  base0=LSB of Input  dbl_ovrd=off  block_type=slice
  slice3 : xbsIndex_r4/Slice  nbits=288  boolean_output=off  mode=Upper Bit Location + Width  bit1=-288  base1=MSB of Input  bit0=0  base0=LSB of Input  dbl_ovrd=off  block_type=slice
  slice4 : xbsIndex_r4/Slice  nbits=288  boolean_output=off  mode=Upper Bit Location + Width  bit1=0  base1=MSB of Input  bit0=0  base0=LSB of Input  dbl_ovrd=off  block_type=slice
  msb_out4 : Outport
  out3 : Outport  Port=2
  out2 : Outport  Port=3
  lsb_out1 : Outport  Port=4
  wires:
  reinterpret1/1 -> lsb_out1/1
  slice1/1 -> reinterpret1/1
  reinterpret2/1 -> out2/1
  slice2/1 -> reinterpret2/1
  reinterpret3/1 -> out3/1
  slice3/1 -> reinterpret3/1
  reinterpret4/1 -> msb_out4/1
  slice4/1 -> reinterpret4/1
  bus_in/1 -> slice1/1, slice2/1, slice3/1, slice4/1
